simulink model "DrivingDistanceD4D5"  (R2018b)
settings: Solver=VariableStepAuto  StartTime=0.0  StopTime=1000  RelTol=1e-3
settings Model: Creator=gregoryseibert  LastModifiedBy=gregoryseibert

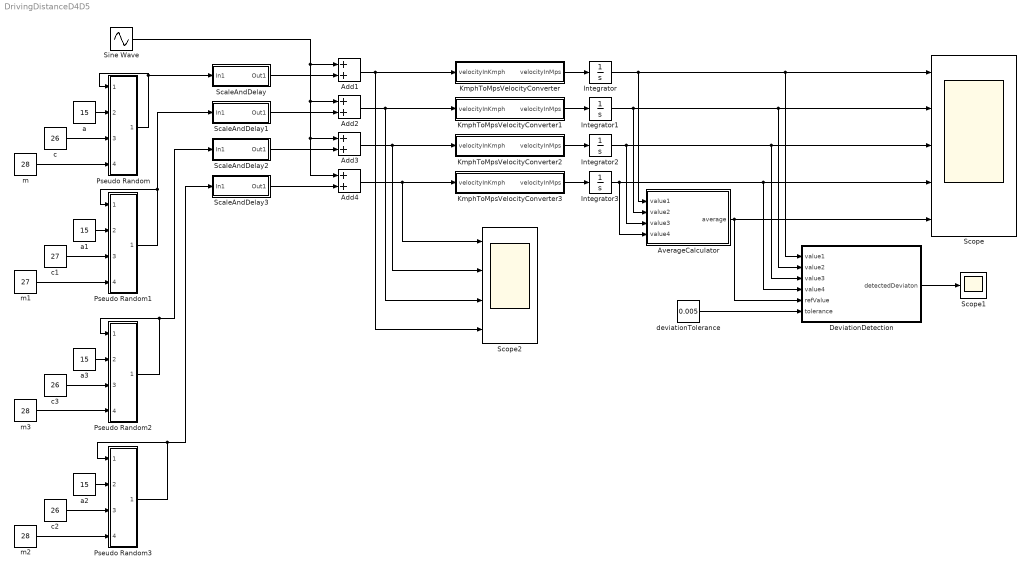
== system DrivingDistanceD4D5 ==
  Add{1..4} (4 alike) : Sum
  AverageCalculator : Subsystem
  DeviationDetection : Subsystem
  Integrator{,1..3} (4 alike) : Integrator
  KmphToMpsVelocityConverter : Subsystem
  KmphToMpsVelocityConverter1 : Subsystem
  KmphToMpsVelocityConverter2 : Subsystem
  KmphToMpsVelocityConverter3 : Subsystem
  Pseudo Random : Subsystem
  Pseudo Random1 : Subsystem
  Pseudo Random2 : Subsystem
  Pseudo Random3 : Subsystem
  ScaleAndDelay : Subsystem
  ScaleAndDelay1 : Subsystem
  ScaleAndDelay2 : Subsystem
  ScaleAndDelay3 : Subsystem
  Scope : Scope  NumInputPorts=5
  Scope1 : Scope
  Scope2 : Scope  NumInputPorts=4
  Sine Wave : Sin  Amplitude=20  SampleTime=0
  a{,1..3} (4 alike) : Constant  Value=15
  c : Constant  Value=26
  c1 : Constant  Value=27
  c2 : Constant  Value=26
  c3 : Constant  Value=26
  deviationTolerance : Constant  Value=0.005
  m : Constant  Value=28
  m1 : Constant  Value=27
  m2 : Constant  Value=28
  m3 : Constant  Value=28
  wires:
  Pseudo Random1/1(Out1) -> ScaleAndDelay1/1(In1), Pseudo Random1/1(In1)
  Pseudo Random3/1(Out1) -> ScaleAndDelay3/1(In1), Pseudo Random3/1(In1)
  Pseudo Random/1(Out1) -> Pseudo Random/1(In1), ScaleAndDelay/1(In1)
  a/1 -> Pseudo Random/2(In2)
  c/1 -> Pseudo Random/3(In3)
  m/1 -> Pseudo Random/4(In4)
  c1/1 -> Pseudo Random1/3(In3)
  a1/1 -> Pseudo Random1/2(In2)
  m1/1 -> Pseudo Random1/4(In4)
  c2/1 -> Pseudo Random3/3(In3)
  a2/1 -> Pseudo Random3/2(In2)
  m2/1 -> Pseudo Random3/4(In4)
  c3/1 -> Pseudo Random2/3(In3)
  Pseudo Random2/1(Out1) -> ScaleAndDelay2/1(In1), Pseudo Random2/1(In1)
  a3/1 -> Pseudo Random2/2(In2)
  m3/1 -> Pseudo Random2/4(In4)
  Sine Wave/1 -> Add4/1, Add3/1, Add2/1, Add1/1
  Integrator2/1 -> AverageCalculator/3(value3), DeviationDetection/3(value3), Scope/3
  KmphToMpsVelocityConverter/1(velocityInMps) -> Integrator/1
  Integrator/1 -> AverageCalculator/1(value1), DeviationDetection/1(value1), Scope/1
  Integrator1/1 -> AverageCalculator/2(value2), DeviationDetection/2(value2), Scope/2
  Integrator3/1 -> AverageCalculator/4(value4), DeviationDetection/4(value4), Scope/4
  KmphToMpsVelocityConverter1/1(velocityInMps) -> Integrator1/1
  Add3/1 -> KmphToMpsVelocityConverter2/1(velocityInKmph), Scope2/2
  KmphToMpsVelocityConverter3/1(velocityInMps) -> Integrator3/1
  Add4/1 -> KmphToMpsVelocityConverter3/1(velocityInKmph), Scope2/1
  deviationTolerance/1 -> DeviationDetection/6(tolerance)
  Add2/1 -> KmphToMpsVelocityConverter1/1(velocityInKmph), Scope2/3
  KmphToMpsVelocityConverter2/1(velocityInMps) -> Integrator2/1
  DeviationDetection/1(detectedDeviaton) -> Scope1/1
  AverageCalculator/1(average) -> DeviationDetection/5(refValue), Scope/5
  Add1/1 -> KmphToMpsVelocityConverter/1(velocityInKmph), Scope2/4
  ScaleAndDelay3/1(Out1) -> Add4/2
  ScaleAndDelay2/1(Out1) -> Add3/2
  ScaleAndDelay1/1(Out1) -> Add2/2
  ScaleAndDelay/1(Out1) -> Add1/2

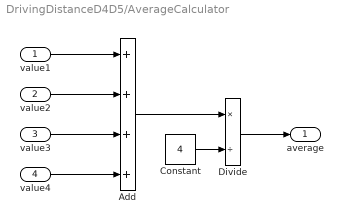
== system DrivingDistanceD4D5/AverageCalculator ==
  value1 : Inport
  value2 : Inport  Port=2
  value3 : Inport  Port=3
  value4 : Inport  Port=4
  Add : Sum  Inputs=++++
  Constant : Constant  Value=4
  Divide : Product  Inputs=*/
  average : Outport
  wires:
  value4/1 -> Add/4
  value3/1 -> Add/3
  Divide/1 -> average/1
  value2/1 -> Add/2
  value1/1 -> Add/1
  Constant/1 -> Divide/2
  Add/1 -> Divide/1

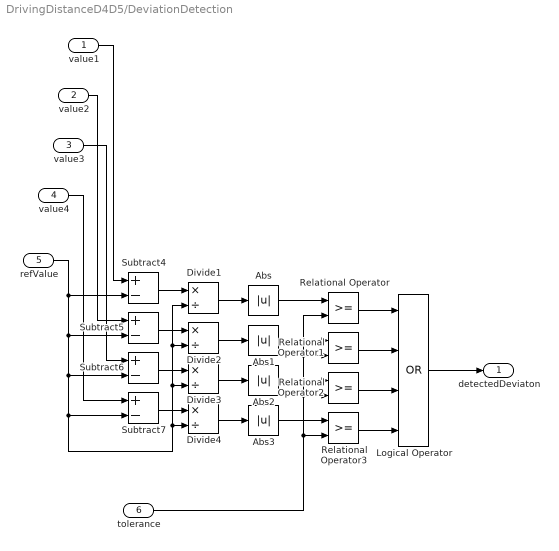
== system DrivingDistanceD4D5/DeviationDetection ==
  value1 : Inport
  value2 : Inport  Port=2
  value3 : Inport  Port=3
  value4 : Inport  Port=4
  refValue : Inport  Port=5
  tolerance : Inport  Port=6
  Abs{,1..3} (4 alike) : Abs
  Divide{1..4} (4 alike) : Product  Inputs=*/
  Logical Operator : Logic  Operator=OR  Inputs=4  AllPortsSameDT=off  OutDataTypeStr=boolean
  Relational Operator{,1..3} (4 alike) : RelationalOperator  OutDataTypeStr=boolean  RndMeth=Simplest
  Subtract{4..7} (4 alike) : Sum  Inputs=+-
  detectedDeviaton : Outport
  wires:
  value1/1 -> Subtract4/1
  Subtract6/1 -> Divide3/1
  Subtract4/1 -> Divide1/1
  Subtract5/1 -> Divide2/1
  Abs1/1 -> Relational Operator1/1
  Logical Operator/1 -> detectedDeviaton/1
  Abs3/1 -> Relational Operator3/1
  Relational Operator/1 -> Logical Operator/1
  Relational Operator1/1 -> Logical Operator/2
  Relational Operator2/1 -> Logical Operator/3
  Divide4/1 -> Abs3/1
  value3/1 -> Subtract6/1
  Divide1/1 -> Abs/1
  value2/1 -> Subtract5/1
  tolerance/1 -> Relational Operator/2, Relational Operator1/2, Relational Operator2/2, Relational Operator3/2
  value4/1 -> Subtract7/1
  Subtract7/1 -> Divide4/1
  Abs/1 -> Relational Operator/1
  Relational Operator3/1 -> Logical Operator/4
  Divide3/1 -> Abs2/1
  Abs2/1 -> Relational Operator2/1
  Divide2/1 -> Abs1/1
  refValue/1 -> Subtract7/2, Divide4/2, Divide3/2, Divide2/2, Divide1/2, Subtract6/2, Subtract5/2, Subtract4/2

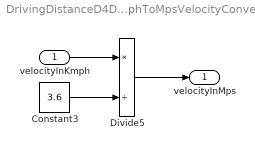
== system DrivingDistanceD4D5/KmphToMpsVelocityConverter ==
  velocityInKmph : Inport
  Constant3 : Constant  Value=3.6
  Divide5 : Product  Inputs=*/
  velocityInMps : Outport
  wires:
  Divide5/1 -> velocityInMps/1
  velocityInKmph/1 -> Divide5/1
  Constant3/1 -> Divide5/2

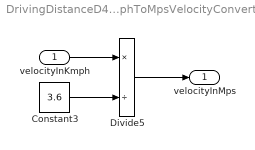
== system DrivingDistanceD4D5/KmphToMpsVelocityConverter1 ==
  velocityInKmph : Inport
  Constant3 : Constant  Value=3.6
  Divide5 : Product  Inputs=*/
  velocityInMps : Outport
  wires:
  Divide5/1 -> velocityInMps/1
  velocityInKmph/1 -> Divide5/1
  Constant3/1 -> Divide5/2

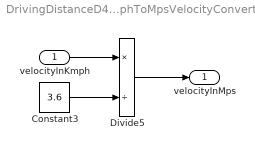
== system DrivingDistanceD4D5/KmphToMpsVelocityConverter2 ==
  velocityInKmph : Inport
  Constant3 : Constant  Value=3.6
  Divide5 : Product  Inputs=*/
  velocityInMps : Outport
  wires:
  Divide5/1 -> velocityInMps/1
  velocityInKmph/1 -> Divide5/1
  Constant3/1 -> Divide5/2

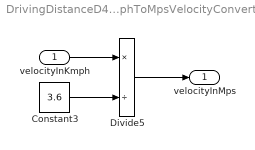
== system DrivingDistanceD4D5/KmphToMpsVelocityConverter3 ==
  velocityInKmph : Inport
  Constant3 : Constant  Value=3.6
  Divide5 : Product  Inputs=*/
  velocityInMps : Outport
  wires:
  Divide5/1 -> velocityInMps/1
  velocityInKmph/1 -> Divide5/1
  Constant3/1 -> Divide5/2

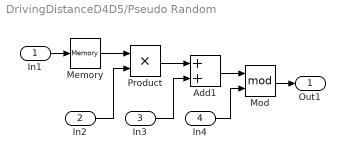
== system DrivingDistanceD4D5/Pseudo Random ==
  In1 : Inport
  In2 : Inport  Port=2
  In3 : Inport  Port=3
  In4 : Inport  Port=4
  Add1 : Sum
  Memory : Memory  InitialCondition=3
  Mod : Math  Operator=mod  SaturateOnIntegerOverflow=on
  Product : Product
  Out1 : Outport
  wires:
  In3/1 -> Add1/2
  In2/1 -> Product/2
  In1/1 -> Memory/1
  In4/1 -> Mod/2
  Memory/1 -> Product/1
  Mod/1 -> Out1/1
  Add1/1 -> Mod/1
  Product/1 -> Add1/1

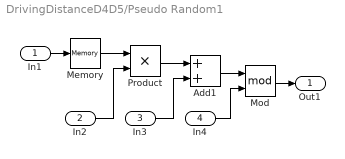
== system DrivingDistanceD4D5/Pseudo Random1 ==
  In1 : Inport
  In2 : Inport  Port=2
  In3 : Inport  Port=3
  In4 : Inport  Port=4
  Add1 : Sum
  Memory : Memory  InitialCondition=3
  Mod : Math  Operator=mod  SaturateOnIntegerOverflow=on
  Product : Product
  Out1 : Outport
  wires:
  In3/1 -> Add1/2
  In2/1 -> Product/2
  In1/1 -> Memory/1
  In4/1 -> Mod/2
  Memory/1 -> Product/1
  Mod/1 -> Out1/1
  Add1/1 -> Mod/1
  Product/1 -> Add1/1

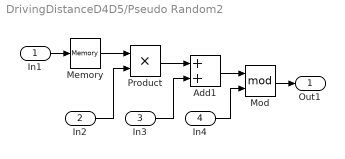
== system DrivingDistanceD4D5/Pseudo Random2 ==
  In1 : Inport
  In2 : Inport  Port=2
  In3 : Inport  Port=3
  In4 : Inport  Port=4
  Add1 : Sum
  Memory : Memory  InitialCondition=3
  Mod : Math  Operator=mod  SaturateOnIntegerOverflow=on
  Product : Product
  Out1 : Outport
  wires:
  In3/1 -> Add1/2
  In2/1 -> Product/2
  In1/1 -> Memory/1
  In4/1 -> Mod/2
  Memory/1 -> Product/1
  Mod/1 -> Out1/1
  Add1/1 -> Mod/1
  Product/1 -> Add1/1

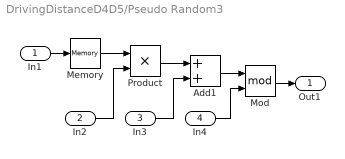
== system DrivingDistanceD4D5/Pseudo Random3 ==
  In1 : Inport
  In2 : Inport  Port=2
  In3 : Inport  Port=3
  In4 : Inport  Port=4
  Add1 : Sum
  Memory : Memory  InitialCondition=3
  Mod : Math  Operator=mod  SaturateOnIntegerOverflow=on
  Product : Product
  Out1 : Outport
  wires:
  In3/1 -> Add1/2
  In2/1 -> Product/2
  In1/1 -> Memory/1
  In4/1 -> Mod/2
  Memory/1 -> Product/1
  Mod/1 -> Out1/1
  Add1/1 -> Mod/1
  Product/1 -> Add1/1

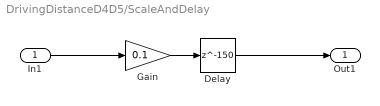
== system DrivingDistanceD4D5/ScaleAndDelay ==
  In1 : Inport
  Delay : Delay  DelayLength=150
  Gain : Gain  Gain=0.1
  Out1 : Outport
  wires:
  Delay/1 -> Out1/1
  In1/1 -> Gain/1
  Gain/1 -> Delay/1

== system DrivingDistanceD4D5/ScaleAndDelay1 ==
  In1 : Inport
  Delay : Delay  DelayLength=150
  Gain : Gain  Gain=0.1
  Out1 : Outport
  wires:
  Delay/1 -> Out1/1
  In1/1 -> Gain/1
  Gain/1 -> Delay/1

== system DrivingDistanceD4D5/ScaleAndDelay2 ==
  In1 : Inport
  Delay : Delay  DelayLength=150
  Gain : Gain  Gain=0.1
  Out1 : Outport
  wires:
  Delay/1 -> Out1/1
  In1/1 -> Gain/1
  Gain/1 -> Delay/1

== system DrivingDistanceD4D5/ScaleAndDelay3 ==
  In1 : Inport
  Delay : Delay  DelayLength=150
  Gain : Gain  Gain=0.1
  Out1 : Outport
  wires:
  Delay/1 -> Out1/1
  In1/1 -> Gain/1
  Gain/1 -> Delay/1
